simulink model "class_5_1C"  (R2023b)
settings: Solver=VariableStepAuto  StartTime=0.0  StopTime=10.0  RelTol=1e-3
values from neighbouring files (symbols this model uses):
  den = [1 2*qsi*wn wn^2]    [class_5_1C.m]
  num = K*wn^2    (= 4)    [class_5_1C.m]
  tSample = 0.1    [class_5_1C.m]
settings Model: Creator=klysm  LastModifiedBy=klysm

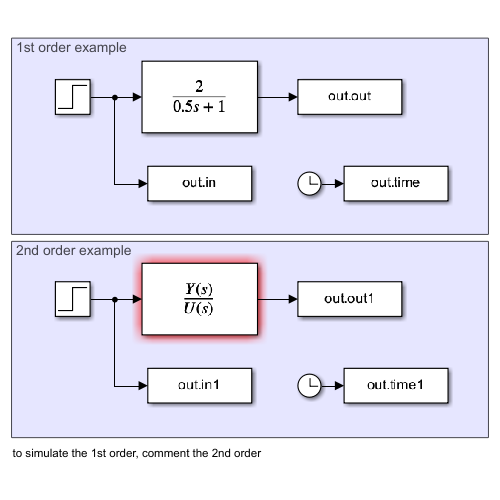
[thumbnail: Simulink's stored preview of the top-level diagram]
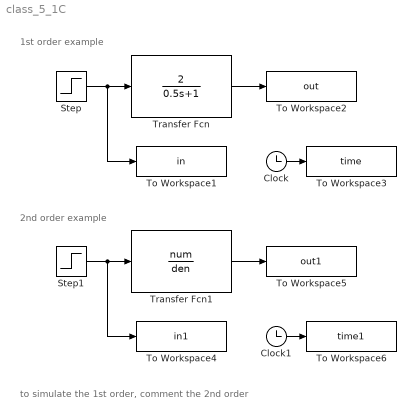
== system class_5_1C ==
  note: to simulate the 1st order, comment the 2nd order
  note: 2nd order example
  note: 1st order example
  Clock : Clock
  Clock1 : Clock
  Step : Step  Time=0  SampleTime=tSample
  Step1 : Step  Time=0  SampleTime=tSample
  To Workspace1 : ToWorkspace  VariableName=in  SampleTime=tSample
  To Workspace2 : ToWorkspace  VariableName=out  SampleTime=tSample
  To Workspace3 : ToWorkspace  VariableName=time  SampleTime=tSample
  To Workspace4 : ToWorkspace  VariableName=in1  SampleTime=tSample
  To Workspace5 : ToWorkspace  VariableName=out1  SampleTime=tSample
  To Workspace6 : ToWorkspace  VariableName=time1  SampleTime=tSample
  Transfer Fcn : TransferFcn  Numerator=2  Denominator=[0.5 1]
  Transfer Fcn1 : TransferFcn  Numerator=num  Denominator=den
  wires:
  Transfer Fcn/1 -> To Workspace2/1
  Step/1 -> To Workspace1/1, Transfer Fcn/1
  Clock/1 -> To Workspace3/1
  Transfer Fcn1/1 -> To Workspace5/1
  Clock1/1 -> To Workspace6/1
  Step1/1 -> To Workspace4/1, Transfer Fcn1/1
